simulink model "space_10"  (R2014b)
settings: Solver=ode45  StartTime=0.0  StopTime=3600000000  RelTol=1e-9
libraries: simulink x1
settings Model: Creator=Tamas  LastModifiedBy=Tamás

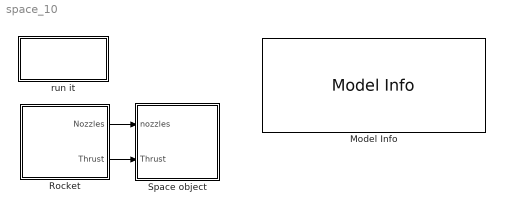
== system space_10 ==
  Model Info : simulink/Model-Wide Utilities/Model Info  Frame=off  DisplayStringWithTags=|  HorizontalTextAlignment=Center  LeftAlignmentValue=0.5  SourceBlockDiagram=space_10  TagMaxNumber=20
      | Model Info
      | Dr. Tamas Szakacs
      | 
      | ModifiedDate 11.10.2020
      | Version: %<ModelVersion>
      | %<Description>
  Rocket : Subsystem
  "Space object " : Subsystem
  run it : Subsystem
      settings: OpenFcn=data_earth_m
      mask Display: disp('Double click to\nload parameters')
  wires:
  Rocket/1(Nozzles) -> "Space object "/1(nozzles)
  Rocket/2(Thrust) -> "Space object "/2(Thrust)

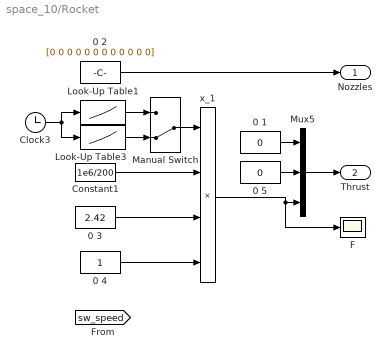
== system space_10/Rocket ==
  0 1 : Constant  Value=0
  0 2 : Constant  Value=[0 0 0 0 0 0 0 0 0 0 0 0]
  0 3 : Constant  Value=2.42
  0 4 : Constant
  0 5 : Constant  Value=0
  Clock3 : Clock
  Constant1 : Constant  Value=1e6/200
  F : Scope
      settings: TimeRange=12  YMax=105  SaveName=ScopeData5
  Look-Up Table1 : Lookup  DialogController=Simulink.DDGSource  InputValues=[0 5322 5323 5522 5523 23870 23870 23870+121 23870+122 70000]  Table=[0 0 1 1 0 0 -1 -1 0 0]  SaturateOnIntegerOverflow=on
  Look-Up Table3 : Lookup  DialogController=Simulink.DDGSource  InputValues=[0 5322 5323 5522 5523 61000 61001 61000+121 61000+122 70000]  Table=[0 0 1 1 0 0 -1 -1 0 0]  SaturateOnIntegerOverflow=on
  Manual Switch : ManualSwitch  CurrentSetting=0
  Mux5 : Mux  Inputs=3
  x_1 : Product  Inputs=****  SaturateOnIntegerOverflow=on  RndMeth=Zero  InputSameDT=on  OutDataTypeStr=Inherit: Same as first input
  Nozzles : Outport
  Thrust : Outport  Port=2
  wires:
  Mux5/1 -> Thrust/1
  Clock3/1 -> Look-Up Table3/1, Look-Up Table1/1
  Look-Up Table3/1 -> Manual Switch/2
  Constant1/1 -> x_1/2
  0 3/1 -> x_1/3
  0 4/1 -> x_1/4
  0 2/1 -> Nozzles/1
  0 5/1 -> Mux5/2
  0 1/1 -> Mux5/1
  x_1/1 -> Mux5/3, F/1
  Manual Switch/1 -> x_1/1
  Look-Up Table1/1 -> Manual Switch/1

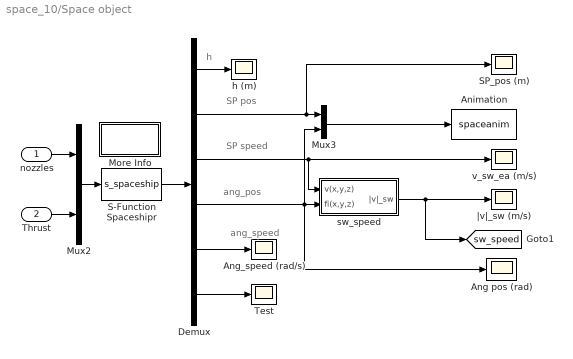
== system space_10/Space object  ==
  note: ang_speed
  note: h
  note: ang_pos
  note: SP pos
  note: SP speed
  nozzles : Inport
  Thrust : Inport  Port=2
  Ang pos (rad) : Scope
      settings: TimeRange=12  YMin=-0.25  YMax=2.75
  "Ang_speed (rad/s)    " : Scope
      settings: TimeRange=12  YMax=105  SaveName=ScopeData3
  "Animation " : S-Function  FunctionName=spaceanim  Parameters=250  EnableBusSupport=off
      settings: DeleteFcn=if ~isempty(findobj('type','figure','name','onecart Animation'));close('onecart Animation'); end;
  Demux : Demux  Outputs=[1 3 3 3 3 3]
  More Info : Subsystem
      mask Display: disp('?')
  Mux2 : Mux  Inputs=[12 3]
  Mux3 : Mux  Inputs=[3 3]
  S-Function Spaceshipr : S-Function  FunctionName=s_spaceship  EnableBusSupport=off
  SP_pos (m) : Scope
      settings: TimeRange=12  YMax=105  SaveName=ScopeData14
  Test : Scope
      settings: TimeRange=10  YMin=0  YMax=1  SaveName=ScopeData17
  h (m) : Scope
      settings: TimeRange=12  YMin=1.21055e+07  YMax=1.33797e+07
  sw_speed : Subsystem
  v_sw_ea (m/s) : Scope
      settings: TimeRange=12  YMin=-0.25  YMax=2.75  SaveName=ScopeData15
  |v|_sw (m/s) : Scope
      settings: TickLabels=on  TimeRange=12  YMin=-0.25  YMax=2.75  SaveName=ScopeData4  SampleInput=on
  tag scope: sw_speed=global
  wires:
  S-Function Spaceshipr/1 -> Demux/1
  Mux2/1 -> S-Function Spaceshipr/1
  Demux/6 -> Test/1
  Demux/3 -> sw_speed/1(v(x,y,z)), v_sw_ea (m/s)/1
  Demux/2 -> SP_pos (m)/1, Mux3/1
  Demux/1 -> h (m)/1
  Demux/5 -> "Ang_speed (rad/s)    "/1
  Mux3/1 -> "Animation "/1
  Demux/4 -> Ang pos (rad)/1, sw_speed/2(fi(x,y,z)), Mux3/2
  nozzles/1 -> Mux2/1
  Thrust/1 -> Mux2/2
  sw_speed/1(|v|_sw) -> [sw_speed], |v|_sw (m/s)/1

== system space_10/run it ==

== system space_10/Space object /More Info ==
  note: Parameters for this unit:
      |
      | parameters_tractor_twotrack.m
      |
      | Last modified at 16.05.2003

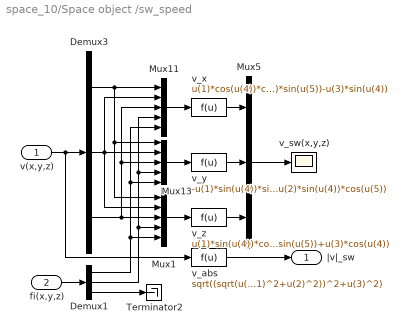
== system space_10/Space object /sw_speed ==
  v(x,y,z) : Inport
  fi(x,y,z) : Inport  Port=2
  Demux1 : Demux  Outputs=3
  Demux3 : Demux  Outputs=3
  Mux1 : Mux  Inputs=5
  Mux11 : Mux  Inputs=5
  Mux13 : Mux  Inputs=5
  Mux5 : Mux  Inputs=3
  Terminator2 : Terminator
  v_abs : Fcn  Expr=sqrt((sqrt(u(1)^2+u(2)^2))^2+u(3)^2)
  v_sw(x,y,z) : Scope
      settings: TimeRange=12  YMin=-0.25  YMax=2.75  SaveName=ScopeData2
  v_x : Fcn  Expr=u(1)*cos(u(4))*cos(u(5))+u(2)*cos(u(4))*sin(u(5))-u(3)*sin(u(4))
  v_y : Fcn  Expr=-u(1)*sin(u(4))*sin(u(5))+u(2)*sin(u(4))*cos(u(5))
  v_z : Fcn  Expr=u(1)*sin(u(4))*cos(u(5))+u(2)*sin(u(4))*sin(u(5))+u(3)*cos(u(4))
  |v|_sw : Outport
  wires:
  Demux3/1 -> Mux1/1, Mux13/1, Mux11/1
  Mux13/1 -> v_y/1
  v_y/1 -> Mux5/2
  Mux5/1 -> v_sw(x,y,z)/1
  v_x/1 -> Mux5/1
  Mux11/1 -> v_x/1
  v(x,y,z)/1 -> v_abs/1, Demux3/1
  Demux3/2 -> Mux1/2, Mux11/2, Mux13/2
  fi(x,y,z)/1 -> Demux1/1
  Demux1/3 -> Terminator2/1
  Mux1/1 -> v_z/1
  v_z/1 -> Mux5/3
  Demux3/3 -> Mux1/3, Mux11/3, Mux13/3
  Demux1/1 -> Mux1/5, Mux13/5, Mux11/5
  Demux1/2 -> Mux13/4, Mux11/4, Mux1/4
  v_abs/1 -> |v|_sw/1
